simulink model "acdcmg_sim8_2_sc_gui"  (R2019b)
settings: Solver=ode8  StartTime=0.0  StopTime=0.5  FixedStep=4e-05  MaxStep=1e-2  RelTol=1e-3
PreLoadFcn:
  | Set_parameters_R2018
InitFcn:
  | Set_parameters_R2018
libraries: opal_lib x23
(part 1 of 2)
settings Model: ARTEMISmethode_block_infos=$$__separator__$$  Creator=Leony  LastModifiedBy=dkh20
settings SolverCC: ZeroCrossAlgorithm=Adaptive  SolverResetMethod=Robust
settings DataIOCC: LimitDataPoints=on  SaveFormat=Array  ReturnWorkspaceOutputs=off
settings OptimizationCC: LocalBlockOutputs=off  LifeSpan=inf
settings DebuggingCC: UnderspecifiedInitializationDetection=Classic  MergeDetectMultiDrivingBlocksExec=none  IgnoredZcDiagnostic=none  SolverPrmCheckMsg=warning  AllowSymbolicDim=off  SFUnexpectedBacktrackingDiag=warning  SFNoUnconditionalDefaultTransitionDiag=warning  SFExecutionAtInitializationDiag=none  ArithmeticOperatorsInVariantConditions=warning
settings HardwareCC: ProdBitPerPointer=32  ProdBitPerSizeT=32  ProdBitPerPtrDiffT=32  ProdLargestAtomicFloat=None  ProdIntDivRoundTo=Undefined  ProdEndianess=Unspecified  ProdWordSize=32  ProdHWDeviceType=32-bit Generic
settings ModelReferenceCC: PropagateSignalLabelsOutOfModel=off
settings SFSimCC: SimUseLocalCustomCode=off  CustomCodeUndefinedFunction=UseInterfaceOnly
settings RTWCC: GenCodeOnly=on  RTWUseLocalCustomCode=off
settings CodeAppCC: StateflowObjectComments=on
settings GRTTargetCC: TargetLangStandard=C89/C90 (ANSI)
settings ConfigComp: CovMetricSettings=dw  CovSaveCumulativeToWorkspaceVar=on  CovSaveSingleToWorkspaceVar=on  CovExternalEMLEnable=off
settings SimscapeCC: SimscapeNormalizeSystem=off

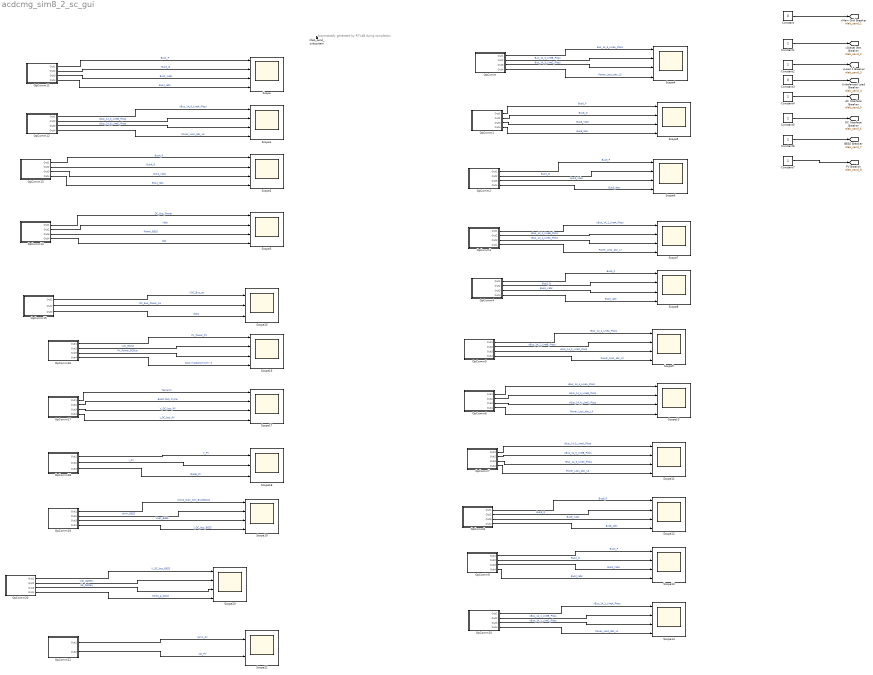
== system acdcmg_sim8_2_sc_gui ==
  note: Automatically generated by RT-LAB during compilation.
  Constant : Constant  Value=0
  Constant{1..2,4..7} (6 alike) : Constant
  Constant3 : Constant  Value=0
  OpComm : Subsystem
      mask init:
      | opmaskdisplay('maskdisplay_block',gcb,'disp(''OpComm'')');
      mask Display:
      | patch([0 0.5 0.7 0],[1 1 0 0],[0.7 0.75 0.9]);
      | patch([1 0.53 0.73 1],[1 1 0 0],[1 0.8 0.7]);
      | plot([0 0 1 1 0],[0 1 1 0 0]);
      | disp('OpComm')
  OpComm1 : Subsystem
      mask init:
      | opmaskdisplay('maskdisplay_block',gcb,'disp(''OpComm'')');
      mask Display:
      | patch([0 0.5 0.7 0],[1 1 0 0],[0.7 0.75 0.9]);
      | patch([1 0.53 0.73 1],[1 1 0 0],[1 0.8 0.7]);
      | plot([0 0 1 1 0],[0 1 1 0 0]);
      | disp('OpComm')
  OpComm10 : Subsystem
      mask init:
      | opmaskdisplay('maskdisplay_block',gcb,'disp(''OpComm'')');
      mask Display:
      | patch([0 0.5 0.7 0],[1 1 0 0],[0.7 0.75 0.9]);
      | patch([1 0.53 0.73 1],[1 1 0 0],[1 0.8 0.7]);
      | plot([0 0 1 1 0],[0 1 1 0 0]);
      | disp('OpComm')
  OpComm11 : Subsystem
      mask init:
      | opmaskdisplay('maskdisplay_block',gcb,'disp(''OpComm'')');
      mask Display:
      | patch([0 0.5 0.7 0],[1 1 0 0],[0.7 0.75 0.9]);
      | patch([1 0.53 0.73 1],[1 1 0 0],[1 0.8 0.7]);
      | plot([0 0 1 1 0],[0 1 1 0 0]);
      | disp('OpComm')
  OpComm12 : Subsystem
      mask init:
      | opmaskdisplay('maskdisplay_block',gcb,'disp(''OpComm'')');
      mask Display:
      | patch([0 0.5 0.7 0],[1 1 0 0],[0.7 0.75 0.9]);
      | patch([1 0.53 0.73 1],[1 1 0 0],[1 0.8 0.7]);
      | plot([0 0 1 1 0],[0 1 1 0 0]);
      | disp('OpComm')
  OpComm13 : Subsystem
      mask init:
      | opmaskdisplay('maskdisplay_block',gcb,'disp(''OpComm'')');
      mask Display:
      | patch([0 0.5 0.7 0],[1 1 0 0],[0.7 0.75 0.9]);
      | patch([1 0.53 0.73 1],[1 1 0 0],[1 0.8 0.7]);
      | plot([0 0 1 1 0],[0 1 1 0 0]);
      | disp('OpComm')
  OpComm14 : Subsystem
      mask init:
      | opmaskdisplay('maskdisplay_block',gcb,'disp(''OpComm'')');
      mask Display:
      | patch([0 0.5 0.7 0],[1 1 0 0],[0.7 0.75 0.9]);
      | patch([1 0.53 0.73 1],[1 1 0 0],[1 0.8 0.7]);
      | plot([0 0 1 1 0],[0 1 1 0 0]);
      | disp('OpComm')
  OpComm15 : Subsystem
      mask init:
      | opmaskdisplay('maskdisplay_block',gcb,'disp(''OpComm'')');
      mask Display:
      | patch([0 0.5 0.7 0],[1 1 0 0],[0.7 0.75 0.9]);
      | patch([1 0.53 0.73 1],[1 1 0 0],[1 0.8 0.7]);
      | plot([0 0 1 1 0],[0 1 1 0 0]);
      | disp('OpComm')
  OpComm16 : Subsystem
      mask init:
      | opmaskdisplay('maskdisplay_block',gcb,'disp(''OpComm'')');
      mask Display:
      | patch([0 0.5 0.7 0],[1 1 0 0],[0.7 0.75 0.9]);
      | patch([1 0.53 0.73 1],[1 1 0 0],[1 0.8 0.7]);
      | plot([0 0 1 1 0],[0 1 1 0 0]);
      | disp('OpComm')
  OpComm17 : Subsystem
      mask init:
      | opmaskdisplay('maskdisplay_block',gcb,'disp(''OpComm'')');
      mask Display:
      | patch([0 0.5 0.7 0],[1 1 0 0],[0.7 0.75 0.9]);
      | patch([1 0.53 0.73 1],[1 1 0 0],[1 0.8 0.7]);
      | plot([0 0 1 1 0],[0 1 1 0 0]);
      | disp('OpComm')
  OpComm18 : Subsystem
      mask init:
      | opmaskdisplay('maskdisplay_block',gcb,'disp(''OpComm'')');
      mask Display:
      | patch([0 0.5 0.7 0],[1 1 0 0],[0.7 0.75 0.9]);
      | patch([1 0.53 0.73 1],[1 1 0 0],[1 0.8 0.7]);
      | plot([0 0 1 1 0],[0 1 1 0 0]);
      | disp('OpComm')
  OpComm19 : Subsystem
      mask init:
      | opmaskdisplay('maskdisplay_block',gcb,'disp(''OpComm'')');
      mask Display:
      | patch([0 0.5 0.7 0],[1 1 0 0],[0.7 0.75 0.9]);
      | patch([1 0.53 0.73 1],[1 1 0 0],[1 0.8 0.7]);
      | plot([0 0 1 1 0],[0 1 1 0 0]);
      | disp('OpComm')
  OpComm2 : Subsystem
      mask init:
      | opmaskdisplay('maskdisplay_block',gcb,'disp(''OpComm'')');
      mask Display:
      | patch([0 0.5 0.7 0],[1 1 0 0],[0.7 0.75 0.9]);
      | patch([1 0.53 0.73 1],[1 1 0 0],[1 0.8 0.7]);
      | plot([0 0 1 1 0],[0 1 1 0 0]);
      | disp('OpComm')
  OpComm20 : Subsystem
      mask init:
      | opmaskdisplay('maskdisplay_block',gcb,'disp(''OpComm'')');
      mask Display:
      | patch([0 0.5 0.7 0],[1 1 0 0],[0.7 0.75 0.9]);
      | patch([1 0.53 0.73 1],[1 1 0 0],[1 0.8 0.7]);
      | plot([0 0 1 1 0],[0 1 1 0 0]);
      | disp('OpComm')
  OpComm21 : Subsystem
      mask init:
      | opmaskdisplay('maskdisplay_block',gcb,'disp(''OpComm'')');
      mask Display:
      | patch([0 0.5 0.7 0],[1 1 0 0],[0.7 0.75 0.9]);
      | patch([1 0.53 0.73 1],[1 1 0 0],[1 0.8 0.7]);
      | plot([0 0 1 1 0],[0 1 1 0 0]);
      | disp('OpComm')
  OpComm3 : Subsystem
      mask init:
      | opmaskdisplay('maskdisplay_block',gcb,'disp(''OpComm'')');
      mask Display:
      | patch([0 0.5 0.7 0],[1 1 0 0],[0.7 0.75 0.9]);
      | patch([1 0.53 0.73 1],[1 1 0 0],[1 0.8 0.7]);
      | plot([0 0 1 1 0],[0 1 1 0 0]);
      | disp('OpComm')
  OpComm4 : Subsystem
      mask init:
      | opmaskdisplay('maskdisplay_block',gcb,'disp(''OpComm'')');
      mask Display:
      | patch([0 0.5 0.7 0],[1 1 0 0],[0.7 0.75 0.9]);
      | patch([1 0.53 0.73 1],[1 1 0 0],[1 0.8 0.7]);
      | plot([0 0 1 1 0],[0 1 1 0 0]);
      | disp('OpComm')
  OpComm5 : Subsystem
      mask init:
      | opmaskdisplay('maskdisplay_block',gcb,'disp(''OpComm'')');
      mask Display:
      | patch([0 0.5 0.7 0],[1 1 0 0],[0.7 0.75 0.9]);
      | patch([1 0.53 0.73 1],[1 1 0 0],[1 0.8 0.7]);
      | plot([0 0 1 1 0],[0 1 1 0 0]);
      | disp('OpComm')
  OpComm6 : Subsystem
      mask init:
      | opmaskdisplay('maskdisplay_block',gcb,'disp(''OpComm'')');
      mask Display:
      | patch([0 0.5 0.7 0],[1 1 0 0],[0.7 0.75 0.9]);
      | patch([1 0.53 0.73 1],[1 1 0 0],[1 0.8 0.7]);
      | plot([0 0 1 1 0],[0 1 1 0 0]);
      | disp('OpComm')
  OpComm7 : Subsystem
      mask init:
      | opmaskdisplay('maskdisplay_block',gcb,'disp(''OpComm'')');
      mask Display:
      | patch([0 0.5 0.7 0],[1 1 0 0],[0.7 0.75 0.9]);
      | patch([1 0.53 0.73 1],[1 1 0 0],[1 0.8 0.7]);
      | plot([0 0 1 1 0],[0 1 1 0 0]);
      | disp('OpComm')
  OpComm8 : Subsystem
      mask init:
      | opmaskdisplay('maskdisplay_block',gcb,'disp(''OpComm'')');
      mask Display:
      | patch([0 0.5 0.7 0],[1 1 0 0],[0.7 0.75 0.9]);
      | patch([1 0.53 0.73 1],[1 1 0 0],[1 0.8 0.7]);
      | plot([0 0 1 1 0],[0 1 1 0 0]);
      | disp('OpComm')
  OpComm9 : Subsystem
      mask init:
      | opmaskdisplay('maskdisplay_block',gcb,'disp(''OpComm'')');
      mask Display:
      | patch([0 0.5 0.7 0],[1 1 0 0],[0.7 0.75 0.9]);
      | patch([1 0.53 0.73 1],[1 1 0 0],[1 0.8 0.7]);
      | plot([0 0 1 1 0],[0 1 1 0 0]);
      | disp('OpComm')
  Scope{,1..14,16..17,19..20} (19 alike) : Scope  NumInputPorts=4
  Scope15 : Scope  NumInputPorts=3
  Scope18 : Scope  NumInputPorts=3
  Scope21 : Scope  NumInputPorts=2
  rtlab_send_subsystem : Subsystem  Priority=-100
      mask Display: text(0,0,'');
  tag scope: rtlab_send_1=global, rtlab_send_2=global, rtlab_send_3=global, rtlab_send_4=global, rtlab_send_5=global, rtlab_send_6=global, rtlab_send_7=global, rtlab_send_8=global
  wires:
  OpComm21/2(Out2) -> Scope21/2  "Idc_PV"
  OpComm21/1(Out1) -> Scope21/1  "Iprim_PV"
  OpComm20/4(Out4) -> Scope20/4  "Comp_g_boost"
  OpComm20/3(Out3) -> Scope20/3  "Idc_battery"
  OpComm20/2(Out2) -> Scope20/2  "Vdc_battery"
  OpComm20/1(Out1) -> Scope20/1  "V_DC_bus_BESS"
  OpComm19/4(Out4) -> Scope19/4  "I_DC_bus_BESS"
  OpComm19/3(Out3) -> Scope19/3  "Vsec_BESS"
  OpComm19/2(Out2) -> Scope19/2  "Iprim_BESS"
  OpComm19/1(Out1) -> Scope19/1  "Comp_Duty_Ctrl_BuckBoost"
  OpComm18/3(Out3) -> Scope18/3  "Idiode_PV"
  OpComm18/2(Out2) -> Scope18/2  "I_PV"
  OpComm18/1(Out1) -> Scope18/1  "V_PV"
  OpComm17/4(Out4) -> Scope17/4  "I_DC_bus_PV"
  OpComm17/3(Out3) -> Scope17/3  "V_DC_bus_PV"
  OpComm17/2(Out2) -> Scope17/2  "Boost Duty Cycle"
  OpComm17/1(Out1) -> Scope17/1  "Temp(C)"
  OpComm16/4(Out4) -> Scope16/4  "Solar Irradiance W/m^2"
  OpComm16/3(Out3) -> Scope16/3  "PV_Power_DCBus"
  OpComm16/2(Out2) -> Scope16/2  "Vdc_Boost"
  OpComm16/1(Out1) -> Scope16/1  "PV_Power_PV"
  OpComm15/3(Out3) -> Scope15/3  "Ibat1"
  OpComm15/2(Out2) -> Scope15/2  "DC_Bus_Power_kw"
  OpComm15/1(Out1) -> Scope15/1  "VDC_Bus_pu"
  OpComm14/4(Out4) -> Scope3/4  "Ibat"
  OpComm14/3(Out3) -> Scope3/3  "Power_BESS"
  OpComm14/2(Out2) -> Scope3/2  "Vbat"
  OpComm14/1(Out1) -> Scope3/1  "DC_Bus_Power"
  OpComm13/4(Out4) -> Scope2/4  "Bus4_Iabc"
  OpComm13/3(Out3) -> Scope2/3  "Bus4_Vabc"
  OpComm13/2(Out2) -> Scope2/2  "Bus4_Q"
  OpComm13/1(Out1) -> Scope2/1  "Bus4_P"
  OpComm12/4(Out4) -> Scope1/4  "Power_Loss_abc_L6"
  OpComm12/3(Out3) -> Scope1/3  "xBus_14_6_LineC_Ploss"
  OpComm12/2(Out2) -> Scope1/2  "xBus_14_6_LineB_Ploss"
  OpComm12/1(Out1) -> Scope1/1  "xBus_14_6_LineA_Ploss"
  OpComm11/4(Out4) -> Scope/4  "Bus1_Iabc"
  OpComm11/3(Out3) -> Scope/3  "Bus1_Vabc"
  OpComm11/2(Out2) -> Scope/2  "Bus1_Q"
  OpComm11/1(Out1) -> Scope/1  "Bus1_P"
  OpComm9/4(Out4) -> Scope13/4  "Bus2_Iabc"
  OpComm9/3(Out3) -> Scope13/3  "Bus2_Vabc"
  OpComm9/2(Out2) -> Scope13/2  "Bus2_Q"
  OpComm9/1(Out1) -> Scope13/1  "Bus2_P"
  OpComm10/4(Out4) -> Scope14/4  "Power_Loss_abc_L1"
  OpComm10/3(Out3) -> Scope14/3  "xBus_14_1_LineC_Ploss"
  OpComm10/2(Out2) -> Scope14/2  "xBus_14_1_LineB_Ploss"
  OpComm10/1(Out1) -> Scope14/1  "xBus_14_1_LineA_Ploss"
  OpComm8/4(Out4) -> Scope12/4  "Bus8_Iabc"
  OpComm8/3(Out3) -> Scope12/3  "Bus8_Vabc"
  OpComm8/2(Out2) -> Scope12/2  "Bus8_Q"
  OpComm8/1(Out1) -> Scope12/1  "Bus8_P"
  OpComm7/4(Out4) -> Scope11/4  "Power_Loss_abc_L5"
  OpComm7/3(Out3) -> Scope11/3  "xBus_14_5_LineC_Ploss"
  OpComm7/2(Out2) -> Scope11/2  "xBus_14_5_LineB_Ploss"
  OpComm7/1(Out1) -> Scope11/1  "xBus_14_5_LineA_Ploss"
  OpComm6/4(Out4) -> Scope10/4  "Power_Loss_abc_L4"
  OpComm6/3(Out3) -> Scope10/3  "xBus_14_4_LineC_Ploss"
  OpComm6/2(Out2) -> Scope10/2  "xBus_14_4_LineB_Ploss"
  OpComm6/1(Out1) -> Scope10/1  "xBus_14_4_LineA_Ploss"
  OpComm5/4(Out4) -> Scope9/4  "Power_Loss_abc_L2"
  OpComm5/3(Out3) -> Scope9/3  "xBus_14_2_LineC_Ploss"
  OpComm5/2(Out2) -> Scope9/2  "xBus_14_2_LineB_Ploss"
  OpComm5/1(Out1) -> Scope9/1  "xBus_14_2_LineA_Ploss"
  OpComm4/1(Out1) -> Scope8/1  "Bus5_P"
  OpComm4/4(Out4) -> Scope8/4  "Bus5_Iabc"
  OpComm4/3(Out3) -> Scope8/3  "Bus5_Vabc"
  OpComm4/2(Out2) -> Scope8/2  "Bus5_Q"
  OpComm3/4(Out4) -> Scope7/4  "Power_Loss_abc_L7"
  OpComm3/1(Out1) -> Scope7/1  "xBus_14_1_LineA_Ploss"
  OpComm3/3(Out3) -> Scope7/3  "xBus_14_1_LineC_Ploss"
  OpComm3/2(Out2) -> Scope7/2  "xBus_14_1_LineB_Ploss"
  OpComm2/4(Out4) -> Scope6/4  "Bus3_Iabc"
  OpComm2/3(Out3) -> Scope6/3  "Bus3_Vabc"
  OpComm2/2(Out2) -> Scope6/2  "Bus3_Q"
  OpComm2/1(Out1) -> Scope6/1  "Bus3_P"
  OpComm1/4(Out4) -> Scope5/4  "Bus6_Iabc"
  OpComm1/1(Out1) -> Scope5/1  "Bus6_P"
  OpComm1/3(Out3) -> Scope5/3  "Bus6_Vabc"
  OpComm1/2(Out2) -> Scope5/2  "Bus6_Q"
  OpComm/4(Out4) -> Scope4/4  "Power_Loss_abc_L3"
  OpComm/3(Out3) -> Scope4/3  "Bus_14_3_LineC_Ploss"
  OpComm/2(Out2) -> Scope4/2  "Bus_14_3_LineB_Ploss"
  OpComm/1(Out1) -> Scope4/1  "Bus_14_3_LineA_Ploss"
  Constant7/1 -> [rtlab_send_8]
  Constant6/1 -> [rtlab_send_7]
  Constant5/1 -> [rtlab_send_6]
  Constant4/1 -> [rtlab_send_5]
  Constant3/1 -> [rtlab_send_4]
  Constant2/1 -> [rtlab_send_3]
  Constant1/1 -> [rtlab_send_2]
  Constant/1 -> [rtlab_send_1]

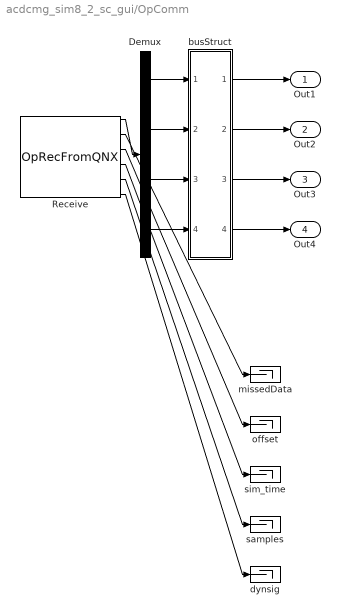
== system acdcmg_sim8_2_sc_gui/OpComm ==
  Demux : Demux  Outputs="[1  1  1  3]"
  Receive : opal_lib/Communication/OpRecFromQNX  Node_num=1  Acqu_Group=1  Data_Width=6  Synchronization=on  Interpolation=on  Threshold=1.0  modelname=ACDCMG_sim8.slx  sampletime=4e-05
  busStruct : Subsystem
  dynsig : Terminator
  missedData : Terminator
  offset : Terminator
  samples : Terminator
  sim_time : Terminator
  Out1 : Outport
  Out2 : Outport  Port=2
  Out3 : Outport  Port=3
  Out4 : Outport  Port=4
  wires:
  Demux/4 -> busStruct/4(In4)
  Demux/3 -> busStruct/3(In3)
  Demux/2 -> busStruct/2(In2)
  Demux/1 -> busStruct/1(In1)
  busStruct/4(Out4) -> Out4/1
  busStruct/3(Out3) -> Out3/1
  busStruct/2(Out2) -> Out2/1
  busStruct/1(Out1) -> Out1/1
  Receive/1 -> Demux/1
  Receive/6 -> dynsig/1
  Receive/5 -> samples/1
  Receive/4 -> sim_time/1
  Receive/3 -> offset/1
  Receive/2 -> missedData/1

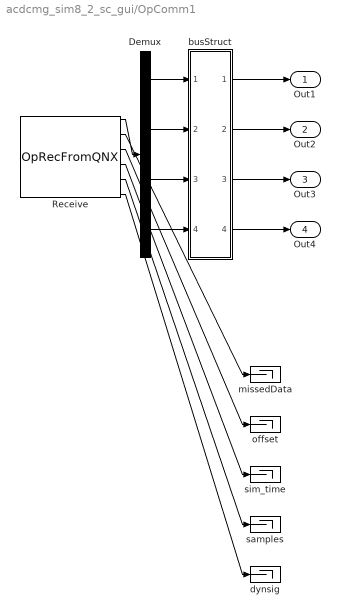
== system acdcmg_sim8_2_sc_gui/OpComm1 ==
  Demux : Demux  Outputs="[1  1  3  3]"
  Receive : opal_lib/Communication/OpRecFromQNX  Node_num=1  Acqu_Group=2  Data_Width=8  Synchronization=on  Interpolation=on  Threshold=1.0  modelname=ACDCMG_sim8.slx  sampletime=4e-05
  busStruct : Subsystem
  dynsig : Terminator
  missedData : Terminator
  offset : Terminator
  samples : Terminator
  sim_time : Terminator
  Out1 : Outport
  Out2 : Outport  Port=2
  Out3 : Outport  Port=3
  Out4 : Outport  Port=4
  wires:
  Demux/4 -> busStruct/4(In4)
  Demux/3 -> busStruct/3(In3)
  Demux/2 -> busStruct/2(In2)
  Demux/1 -> busStruct/1(In1)
  busStruct/4(Out4) -> Out4/1
  busStruct/3(Out3) -> Out3/1
  busStruct/2(Out2) -> Out2/1
  busStruct/1(Out1) -> Out1/1
  Receive/1 -> Demux/1
  Receive/6 -> dynsig/1
  Receive/5 -> samples/1
  Receive/4 -> sim_time/1
  Receive/3 -> offset/1
  Receive/2 -> missedData/1

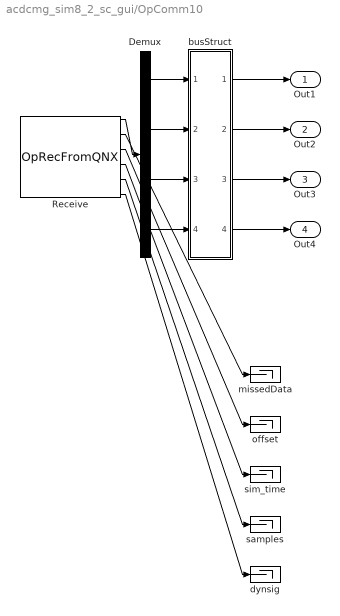
== system acdcmg_sim8_2_sc_gui/OpComm10 ==
  Demux : Demux  Outputs="[1  1  1  3]"
  Receive : opal_lib/Communication/OpRecFromQNX  Node_num=1  Acqu_Group=11  Data_Width=6  Synchronization=on  Interpolation=on  Threshold=1.0  modelname=ACDCMG_sim8.slx  sampletime=4e-05
  busStruct : Subsystem
  dynsig : Terminator
  missedData : Terminator
  offset : Terminator
  samples : Terminator
  sim_time : Terminator
  Out1 : Outport
  Out2 : Outport  Port=2
  Out3 : Outport  Port=3
  Out4 : Outport  Port=4
  wires:
  Demux/4 -> busStruct/4(In4)
  Demux/3 -> busStruct/3(In3)
  Demux/2 -> busStruct/2(In2)
  Demux/1 -> busStruct/1(In1)
  busStruct/4(Out4) -> Out4/1
  busStruct/3(Out3) -> Out3/1
  busStruct/2(Out2) -> Out2/1
  busStruct/1(Out1) -> Out1/1
  Receive/1 -> Demux/1
  Receive/6 -> dynsig/1
  Receive/5 -> samples/1
  Receive/4 -> sim_time/1
  Receive/3 -> offset/1
  Receive/2 -> missedData/1

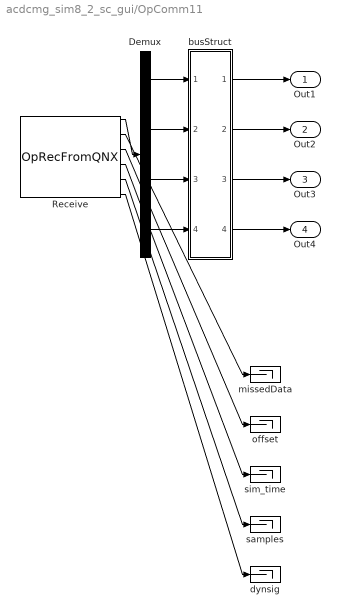
== system acdcmg_sim8_2_sc_gui/OpComm11 ==
  Demux : Demux  Outputs="[1  1  3  3]"
  Receive : opal_lib/Communication/OpRecFromQNX  Node_num=1  Acqu_Group=12  Data_Width=8  Synchronization=on  Interpolation=on  Threshold=1.0  modelname=ACDCMG_sim8.slx  sampletime=4e-05
  busStruct : Subsystem
  dynsig : Terminator
  missedData : Terminator
  offset : Terminator
  samples : Terminator
  sim_time : Terminator
  Out1 : Outport
  Out2 : Outport  Port=2
  Out3 : Outport  Port=3
  Out4 : Outport  Port=4
  wires:
  Demux/4 -> busStruct/4(In4)
  Demux/3 -> busStruct/3(In3)
  Demux/2 -> busStruct/2(In2)
  Demux/1 -> busStruct/1(In1)
  busStruct/4(Out4) -> Out4/1
  busStruct/3(Out3) -> Out3/1
  busStruct/2(Out2) -> Out2/1
  busStruct/1(Out1) -> Out1/1
  Receive/1 -> Demux/1
  Receive/6 -> dynsig/1
  Receive/5 -> samples/1
  Receive/4 -> sim_time/1
  Receive/3 -> offset/1
  Receive/2 -> missedData/1

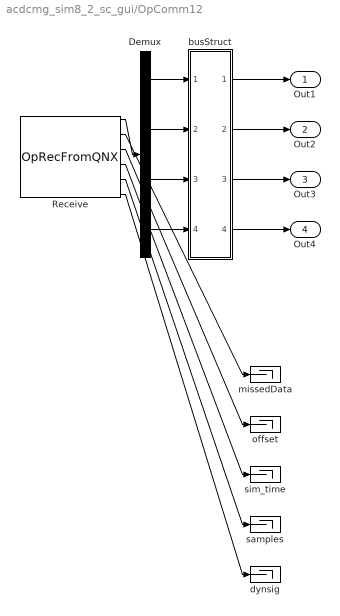
== system acdcmg_sim8_2_sc_gui/OpComm12 ==
  Demux : Demux  Outputs="[1  1  1  3]"
  Receive : opal_lib/Communication/OpRecFromQNX  Node_num=1  Acqu_Group=13  Data_Width=6  Synchronization=on  Interpolation=on  Threshold=1.0  modelname=ACDCMG_sim8.slx  sampletime=4e-05
  busStruct : Subsystem
  dynsig : Terminator
  missedData : Terminator
  offset : Terminator
  samples : Terminator
  sim_time : Terminator
  Out1 : Outport
  Out2 : Outport  Port=2
  Out3 : Outport  Port=3
  Out4 : Outport  Port=4
  wires:
  Demux/4 -> busStruct/4(In4)
  Demux/3 -> busStruct/3(In3)
  Demux/2 -> busStruct/2(In2)
  Demux/1 -> busStruct/1(In1)
  busStruct/4(Out4) -> Out4/1
  busStruct/3(Out3) -> Out3/1
  busStruct/2(Out2) -> Out2/1
  busStruct/1(Out1) -> Out1/1
  Receive/1 -> Demux/1
  Receive/6 -> dynsig/1
  Receive/5 -> samples/1
  Receive/4 -> sim_time/1
  Receive/3 -> offset/1
  Receive/2 -> missedData/1

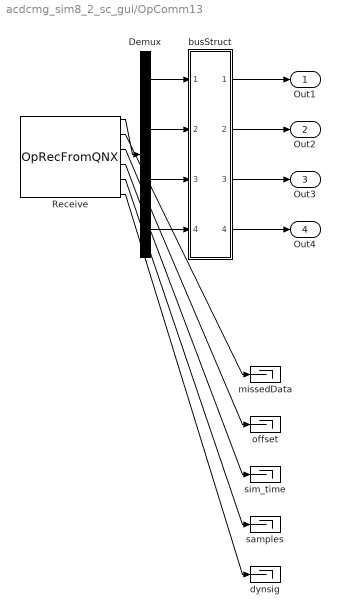
== system acdcmg_sim8_2_sc_gui/OpComm13 ==
  Demux : Demux  Outputs="[1  1  3  3]"
  Receive : opal_lib/Communication/OpRecFromQNX  Node_num=1  Acqu_Group=14  Data_Width=8  Synchronization=on  Interpolation=on  Threshold=1.0  modelname=ACDCMG_sim8.slx  sampletime=4e-05
  busStruct : Subsystem
  dynsig : Terminator
  missedData : Terminator
  offset : Terminator
  samples : Terminator
  sim_time : Terminator
  Out1 : Outport
  Out2 : Outport  Port=2
  Out3 : Outport  Port=3
  Out4 : Outport  Port=4
  wires:
  Demux/4 -> busStruct/4(In4)
  Demux/3 -> busStruct/3(In3)
  Demux/2 -> busStruct/2(In2)
  Demux/1 -> busStruct/1(In1)
  busStruct/4(Out4) -> Out4/1
  busStruct/3(Out3) -> Out3/1
  busStruct/2(Out2) -> Out2/1
  busStruct/1(Out1) -> Out1/1
  Receive/1 -> Demux/1
  Receive/6 -> dynsig/1
  Receive/5 -> samples/1
  Receive/4 -> sim_time/1
  Receive/3 -> offset/1
  Receive/2 -> missedData/1

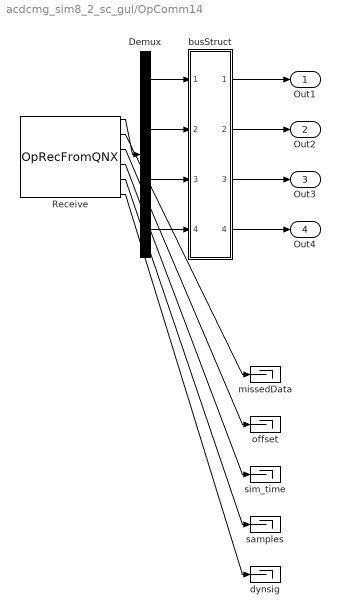
== system acdcmg_sim8_2_sc_gui/OpComm14 ==
  Demux : Demux  Outputs="[1  1  1  1]"
  Receive : opal_lib/Communication/OpRecFromQNX  Node_num=1  Acqu_Group=16  Data_Width=4  Synchronization=on  Interpolation=on  Threshold=1.0  modelname=ACDCMG_sim8.slx  sampletime=4e-05
  busStruct : Subsystem
  dynsig : Terminator
  missedData : Terminator
  offset : Terminator
  samples : Terminator
  sim_time : Terminator
  Out1 : Outport
  Out2 : Outport  Port=2
  Out3 : Outport  Port=3
  Out4 : Outport  Port=4
  wires:
  Demux/4 -> busStruct/4(In4)
  Demux/3 -> busStruct/3(In3)
  Demux/2 -> busStruct/2(In2)
  Demux/1 -> busStruct/1(In1)
  busStruct/4(Out4) -> Out4/1
  busStruct/3(Out3) -> Out3/1
  busStruct/2(Out2) -> Out2/1
  busStruct/1(Out1) -> Out1/1
  Receive/1 -> Demux/1
  Receive/6 -> dynsig/1
  Receive/5 -> samples/1
  Receive/4 -> sim_time/1
  Receive/3 -> offset/1
  Receive/2 -> missedData/1

== system acdcmg_sim8_2_sc_gui/OpComm15 ==
  Demux : Demux  Outputs="[1  1  1]"
  Receive : opal_lib/Communication/OpRecFromQNX  Node_num=1  Acqu_Group=17  Data_Width=3  Synchronization=on  Interpolation=on  Threshold=1.0  modelname=ACDCMG_sim8.slx  sampletime=4e-05
  busStruct : Subsystem
  dynsig : Terminator
  missedData : Terminator
  offset : Terminator
  samples : Terminator
  sim_time : Terminator
  Out1 : Outport
  Out2 : Outport  Port=2
  Out3 : Outport  Port=3
  wires:
  Demux/3 -> busStruct/3(In3)
  Demux/2 -> busStruct/2(In2)
  Demux/1 -> busStruct/1(In1)
  busStruct/3(Out3) -> Out3/1
  busStruct/2(Out2) -> Out2/1
  busStruct/1(Out1) -> Out1/1
  Receive/1 -> Demux/1
  Receive/6 -> dynsig/1
  Receive/5 -> samples/1
  Receive/4 -> sim_time/1
  Receive/3 -> offset/1
  Receive/2 -> missedData/1

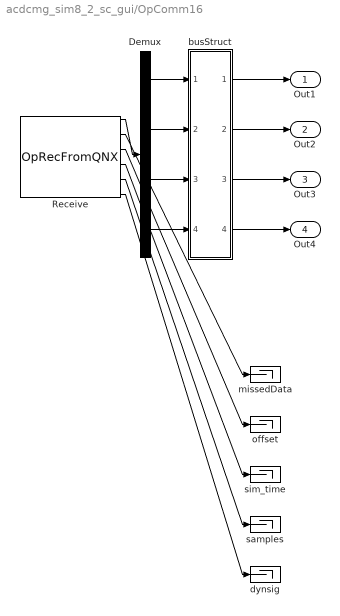
== system acdcmg_sim8_2_sc_gui/OpComm16 ==
  Demux : Demux  Outputs="[1  1  1  1]"
  Receive : opal_lib/Communication/OpRecFromQNX  Node_num=1  Acqu_Group=18  Data_Width=4  Synchronization=on  Interpolation=on  Threshold=1.0  modelname=ACDCMG_sim8.slx  sampletime=4e-05
  busStruct : Subsystem
  dynsig : Terminator
  missedData : Terminator
  offset : Terminator
  samples : Terminator
  sim_time : Terminator
  Out1 : Outport
  Out2 : Outport  Port=2
  Out3 : Outport  Port=3
  Out4 : Outport  Port=4
  wires:
  Demux/4 -> busStruct/4(In4)
  Demux/3 -> busStruct/3(In3)
  Demux/2 -> busStruct/2(In2)
  Demux/1 -> busStruct/1(In1)
  busStruct/4(Out4) -> Out4/1
  busStruct/3(Out3) -> Out3/1
  busStruct/2(Out2) -> Out2/1
  busStruct/1(Out1) -> Out1/1
  Receive/1 -> Demux/1
  Receive/6 -> dynsig/1
  Receive/5 -> samples/1
  Receive/4 -> sim_time/1
  Receive/3 -> offset/1
  Receive/2 -> missedData/1

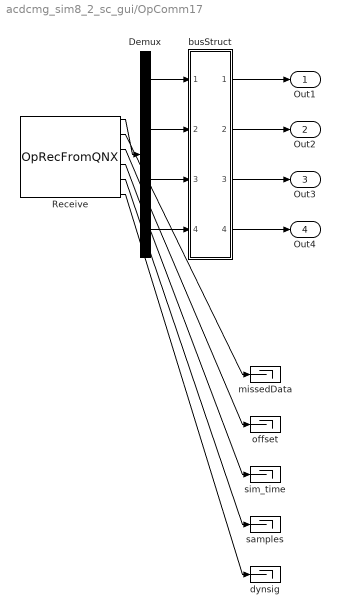
== system acdcmg_sim8_2_sc_gui/OpComm17 ==
  Demux : Demux  Outputs="[1  1  1  1]"
  Receive : opal_lib/Communication/OpRecFromQNX  Node_num=1  Acqu_Group=19  Data_Width=4  Synchronization=on  Interpolation=on  Threshold=1.0  modelname=ACDCMG_sim8.slx  sampletime=4e-05
  busStruct : Subsystem
  dynsig : Terminator
  missedData : Terminator
  offset : Terminator
  samples : Terminator
  sim_time : Terminator
  Out1 : Outport
  Out2 : Outport  Port=2
  Out3 : Outport  Port=3
  Out4 : Outport  Port=4
  wires:
  Demux/4 -> busStruct/4(In4)
  Demux/3 -> busStruct/3(In3)
  Demux/2 -> busStruct/2(In2)
  Demux/1 -> busStruct/1(In1)
  busStruct/4(Out4) -> Out4/1
  busStruct/3(Out3) -> Out3/1
  busStruct/2(Out2) -> Out2/1
  busStruct/1(Out1) -> Out1/1
  Receive/1 -> Demux/1
  Receive/6 -> dynsig/1
  Receive/5 -> samples/1
  Receive/4 -> sim_time/1
  Receive/3 -> offset/1
  Receive/2 -> missedData/1

== system acdcmg_sim8_2_sc_gui/OpComm18 ==
  Demux : Demux  Outputs="[1  1  1]"
  Receive : opal_lib/Communication/OpRecFromQNX  Node_num=1  Acqu_Group=20  Data_Width=3  Synchronization=on  Interpolation=on  Threshold=1.0  modelname=ACDCMG_sim8.slx  sampletime=4e-05
  busStruct : Subsystem
  dynsig : Terminator
  missedData : Terminator
  offset : Terminator
  samples : Terminator
  sim_time : Terminator
  Out1 : Outport
  Out2 : Outport  Port=2
  Out3 : Outport  Port=3
  wires:
  Demux/3 -> busStruct/3(In3)
  Demux/2 -> busStruct/2(In2)
  Demux/1 -> busStruct/1(In1)
  busStruct/3(Out3) -> Out3/1
  busStruct/2(Out2) -> Out2/1
  busStruct/1(Out1) -> Out1/1
  Receive/1 -> Demux/1
  Receive/6 -> dynsig/1
  Receive/5 -> samples/1
  Receive/4 -> sim_time/1
  Receive/3 -> offset/1
  Receive/2 -> missedData/1

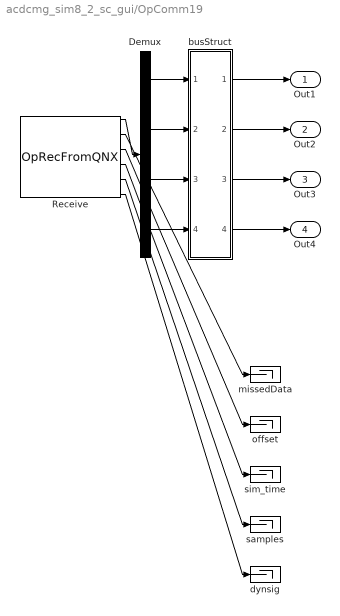
== system acdcmg_sim8_2_sc_gui/OpComm19 ==
  Demux : Demux  Outputs="[1  1  1  1]"
  Receive : opal_lib/Communication/OpRecFromQNX  Node_num=1  Acqu_Group=21  Data_Width=4  Synchronization=on  Interpolation=on  Threshold=1.0  modelname=ACDCMG_sim8.slx  sampletime=4e-05
  busStruct : Subsystem
  dynsig : Terminator
  missedData : Terminator
  offset : Terminator
  samples : Terminator
  sim_time : Terminator
  Out1 : Outport
  Out2 : Outport  Port=2
  Out3 : Outport  Port=3
  Out4 : Outport  Port=4
  wires:
  Demux/4 -> busStruct/4(In4)
  Demux/3 -> busStruct/3(In3)
  Demux/2 -> busStruct/2(In2)
  Demux/1 -> busStruct/1(In1)
  busStruct/4(Out4) -> Out4/1
  busStruct/3(Out3) -> Out3/1
  busStruct/2(Out2) -> Out2/1
  busStruct/1(Out1) -> Out1/1
  Receive/1 -> Demux/1
  Receive/6 -> dynsig/1
  Receive/5 -> samples/1
  Receive/4 -> sim_time/1
  Receive/3 -> offset/1
  Receive/2 -> missedData/1

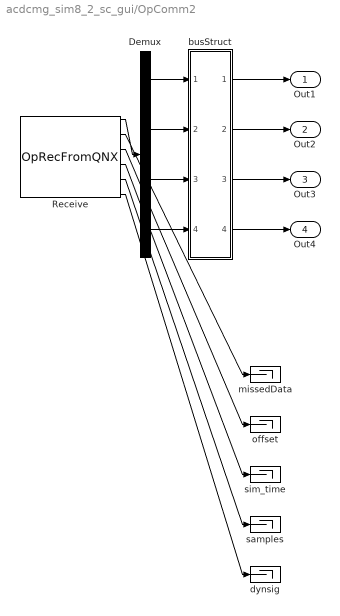
== system acdcmg_sim8_2_sc_gui/OpComm2 ==
  Demux : Demux  Outputs="[1  1  3  3]"
  Receive : opal_lib/Communication/OpRecFromQNX  Node_num=1  Acqu_Group=3  Data_Width=8  Synchronization=on  Interpolation=on  Threshold=1.0  modelname=ACDCMG_sim8.slx  sampletime=4e-05
  busStruct : Subsystem
  dynsig : Terminator
  missedData : Terminator
  offset : Terminator
  samples : Terminator
  sim_time : Terminator
  Out1 : Outport
  Out2 : Outport  Port=2
  Out3 : Outport  Port=3
  Out4 : Outport  Port=4
  wires:
  Demux/4 -> busStruct/4(In4)
  Demux/3 -> busStruct/3(In3)
  Demux/2 -> busStruct/2(In2)
  Demux/1 -> busStruct/1(In1)
  busStruct/4(Out4) -> Out4/1
  busStruct/3(Out3) -> Out3/1
  busStruct/2(Out2) -> Out2/1
  busStruct/1(Out1) -> Out1/1
  Receive/1 -> Demux/1
  Receive/6 -> dynsig/1
  Receive/5 -> samples/1
  Receive/4 -> sim_time/1
  Receive/3 -> offset/1
  Receive/2 -> missedData/1

== system acdcmg_sim8_2_sc_gui/OpComm20 ==
  Demux : Demux  Outputs="[1  1  1  1]"
  Receive : opal_lib/Communication/OpRecFromQNX  Node_num=1  Acqu_Group=22  Data_Width=4  Synchronization=on  Interpolation=on  Threshold=1.0  modelname=ACDCMG_sim8.slx  sampletime=4e-05
  busStruct : Subsystem
  dynsig : Terminator
  missedData : Terminator
  offset : Terminator
  samples : Terminator
  sim_time : Terminator
  Out1 : Outport
  Out2 : Outport  Port=2
  Out3 : Outport  Port=3
  Out4 : Outport  Port=4
  wires:
  Demux/4 -> busStruct/4(In4)
  Demux/3 -> busStruct/3(In3)
  Demux/2 -> busStruct/2(In2)
  Demux/1 -> busStruct/1(In1)
  busStruct/4(Out4) -> Out4/1
  busStruct/3(Out3) -> Out3/1
  busStruct/2(Out2) -> Out2/1
  busStruct/1(Out1) -> Out1/1
  Receive/1 -> Demux/1
  Receive/6 -> dynsig/1
  Receive/5 -> samples/1
  Receive/4 -> sim_time/1
  Receive/3 -> offset/1
  Receive/2 -> missedData/1

== system acdcmg_sim8_2_sc_gui/OpComm21 ==
  Demux : Demux  Outputs="[1  1]"
  Receive : opal_lib/Communication/OpRecFromQNX  Node_num=1  Acqu_Group=23  Data_Width=2  Synchronization=on  Interpolation=on  Threshold=1.0  modelname=ACDCMG_sim8.slx  sampletime=4e-05
  busStruct : Subsystem
  dynsig : Terminator
  missedData : Terminator
  offset : Terminator
  samples : Terminator
  sim_time : Terminator
  Out1 : Outport
  Out2 : Outport  Port=2
  wires:
  Demux/2 -> busStruct/2(In2)
  Demux/1 -> busStruct/1(In1)
  busStruct/2(Out2) -> Out2/1
  busStruct/1(Out1) -> Out1/1
  Receive/1 -> Demux/1
  Receive/6 -> dynsig/1
  Receive/5 -> samples/1
  Receive/4 -> sim_time/1
  Receive/3 -> offset/1
  Receive/2 -> missedData/1

== system acdcmg_sim8_2_sc_gui/OpComm3 ==
  Demux : Demux  Outputs="[1  1  1  3]"
  Receive : opal_lib/Communication/OpRecFromQNX  Node_num=1  Acqu_Group=4  Data_Width=6  Synchronization=on  Interpolation=on  Threshold=1.0  modelname=ACDCMG_sim8.slx  sampletime=4e-05
  busStruct : Subsystem
  dynsig : Terminator
  missedData : Terminator
  offset : Terminator
  samples : Terminator
  sim_time : Terminator
  Out1 : Outport
  Out2 : Outport  Port=2
  Out3 : Outport  Port=3
  Out4 : Outport  Port=4
  wires:
  Demux/4 -> busStruct/4(In4)
  Demux/3 -> busStruct/3(In3)
  Demux/2 -> busStruct/2(In2)
  Demux/1 -> busStruct/1(In1)
  busStruct/4(Out4) -> Out4/1
  busStruct/3(Out3) -> Out3/1
  busStruct/2(Out2) -> Out2/1
  busStruct/1(Out1) -> Out1/1
  Receive/1 -> Demux/1
  Receive/6 -> dynsig/1
  Receive/5 -> samples/1
  Receive/4 -> sim_time/1
  Receive/3 -> offset/1
  Receive/2 -> missedData/1

== system acdcmg_sim8_2_sc_gui/OpComm4 ==
  Demux : Demux  Outputs="[1  1  4  3]"
  Receive : opal_lib/Communication/OpRecFromQNX  Node_num=1  Acqu_Group=5  Data_Width=9  Synchronization=on  Interpolation=on  Threshold=1.0  modelname=ACDCMG_sim8.slx  sampletime=4e-05
  busStruct : Subsystem
  dynsig : Terminator
  missedData : Terminator
  offset : Terminator
  samples : Terminator
  sim_time : Terminator
  Out1 : Outport
  Out2 : Outport  Port=2
  Out3 : Outport  Port=3
  Out4 : Outport  Port=4
  wires:
  Demux/4 -> busStruct/4(In4)
  Demux/3 -> busStruct/3(In3)
  Demux/2 -> busStruct/2(In2)
  Demux/1 -> busStruct/1(In1)
  busStruct/4(Out4) -> Out4/1
  busStruct/3(Out3) -> Out3/1
  busStruct/2(Out2) -> Out2/1
  busStruct/1(Out1) -> Out1/1
  Receive/1 -> Demux/1
  Receive/6 -> dynsig/1
  Receive/5 -> samples/1
  Receive/4 -> sim_time/1
  Receive/3 -> offset/1
  Receive/2 -> missedData/1

== system acdcmg_sim8_2_sc_gui/OpComm5 ==
  Demux : Demux  Outputs="[1  1  1  3]"
  Receive : opal_lib/Communication/OpRecFromQNX  Node_num=1  Acqu_Group=6  Data_Width=6  Synchronization=on  Interpolation=on  Threshold=1.0  modelname=ACDCMG_sim8.slx  sampletime=4e-05
  busStruct : Subsystem
  dynsig : Terminator
  missedData : Terminator
  offset : Terminator
  samples : Terminator
  sim_time : Terminator
  Out1 : Outport
  Out2 : Outport  Port=2
  Out3 : Outport  Port=3
  Out4 : Outport  Port=4
  wires:
  Demux/4 -> busStruct/4(In4)
  Demux/3 -> busStruct/3(In3)
  Demux/2 -> busStruct/2(In2)
  Demux/1 -> busStruct/1(In1)
  busStruct/4(Out4) -> Out4/1
  busStruct/3(Out3) -> Out3/1
  busStruct/2(Out2) -> Out2/1
  busStruct/1(Out1) -> Out1/1
  Receive/1 -> Demux/1
  Receive/6 -> dynsig/1
  Receive/5 -> samples/1
  Receive/4 -> sim_time/1
  Receive/3 -> offset/1
  Receive/2 -> missedData/1

== system acdcmg_sim8_2_sc_gui/OpComm6 ==
  Demux : Demux  Outputs="[1  1  1  3]"
  Receive : opal_lib/Communication/OpRecFromQNX  Node_num=1  Acqu_Group=7  Data_Width=6  Synchronization=on  Interpolation=on  Threshold=1.0  modelname=ACDCMG_sim8.slx  sampletime=4e-05
  busStruct : Subsystem
  dynsig : Terminator
  missedData : Terminator
  offset : Terminator
  samples : Terminator
  sim_time : Terminator
  Out1 : Outport
  Out2 : Outport  Port=2
  Out3 : Outport  Port=3
  Out4 : Outport  Port=4
  wires:
  Demux/4 -> busStruct/4(In4)
  Demux/3 -> busStruct/3(In3)
  Demux/2 -> busStruct/2(In2)
  Demux/1 -> busStruct/1(In1)
  busStruct/4(Out4) -> Out4/1
  busStruct/3(Out3) -> Out3/1
  busStruct/2(Out2) -> Out2/1
  busStruct/1(Out1) -> Out1/1
  Receive/1 -> Demux/1
  Receive/6 -> dynsig/1
  Receive/5 -> samples/1
  Receive/4 -> sim_time/1
  Receive/3 -> offset/1
  Receive/2 -> missedData/1

== system acdcmg_sim8_2_sc_gui/OpComm7 ==
  Demux : Demux  Outputs="[1  1  1  3]"
  Receive : opal_lib/Communication/OpRecFromQNX  Node_num=1  Acqu_Group=8  Data_Width=6  Synchronization=on  Interpolation=on  Threshold=1.0  modelname=ACDCMG_sim8.slx  sampletime=4e-05
  busStruct : Subsystem
  dynsig : Terminator
  missedData : Terminator
  offset : Terminator
  samples : Terminator
  sim_time : Terminator
  Out1 : Outport
  Out2 : Outport  Port=2
  Out3 : Outport  Port=3
  Out4 : Outport  Port=4
  wires:
  Demux/4 -> busStruct/4(In4)
  Demux/3 -> busStruct/3(In3)
  Demux/2 -> busStruct/2(In2)
  Demux/1 -> busStruct/1(In1)
  busStruct/4(Out4) -> Out4/1
  busStruct/3(Out3) -> Out3/1
  busStruct/2(Out2) -> Out2/1
  busStruct/1(Out1) -> Out1/1
  Receive/1 -> Demux/1
  Receive/6 -> dynsig/1
  Receive/5 -> samples/1
  Receive/4 -> sim_time/1
  Receive/3 -> offset/1
  Receive/2 -> missedData/1

== system acdcmg_sim8_2_sc_gui/OpComm8 ==
  Demux : Demux  Outputs="[1  1  3  3]"
  Receive : opal_lib/Communication/OpRecFromQNX  Node_num=1  Acqu_Group=9  Data_Width=8  Synchronization=on  Interpolation=on  Threshold=1.0  modelname=ACDCMG_sim8.slx  sampletime=4e-05
  busStruct : Subsystem
  dynsig : Terminator
  missedData : Terminator
  offset : Terminator
  samples : Terminator
  sim_time : Terminator
  Out1 : Outport
  Out2 : Outport  Port=2
  Out3 : Outport  Port=3
  Out4 : Outport  Port=4
  wires:
  Demux/4 -> busStruct/4(In4)
  Demux/3 -> busStruct/3(In3)
  Demux/2 -> busStruct/2(In2)
  Demux/1 -> busStruct/1(In1)
  busStruct/4(Out4) -> Out4/1
  busStruct/3(Out3) -> Out3/1
  busStruct/2(Out2) -> Out2/1
  busStruct/1(Out1) -> Out1/1
  Receive/1 -> Demux/1
  Receive/6 -> dynsig/1
  Receive/5 -> samples/1
  Receive/4 -> sim_time/1
  Receive/3 -> offset/1
  Receive/2 -> missedData/1

== system acdcmg_sim8_2_sc_gui/OpComm9 ==
  Demux : Demux  Outputs="[1  1  3  3]"
  Receive : opal_lib/Communication/OpRecFromQNX  Node_num=1  Acqu_Group=10  Data_Width=8  Synchronization=on  Interpolation=on  Threshold=1.0  modelname=ACDCMG_sim8.slx  sampletime=4e-05
  busStruct : Subsystem
  dynsig : Terminator
  missedData : Terminator
  offset : Terminator
  samples : Terminator
  sim_time : Terminator
  Out1 : Outport
  Out2 : Outport  Port=2
  Out3 : Outport  Port=3
  Out4 : Outport  Port=4
  wires:
  Demux/4 -> busStruct/4(In4)
  Demux/3 -> busStruct/3(In3)
  Demux/2 -> busStruct/2(In2)
  Demux/1 -> busStruct/1(In1)
  busStruct/4(Out4) -> Out4/1
  busStruct/3(Out3) -> Out3/1
  busStruct/2(Out2) -> Out2/1
  busStruct/1(Out1) -> Out1/1
  Receive/1 -> Demux/1
  Receive/6 -> dynsig/1
  Receive/5 -> samples/1
  Receive/4 -> sim_time/1
  Receive/3 -> offset/1
  Receive/2 -> missedData/1

== system acdcmg_sim8_2_sc_gui/rtlab_send_subsystem ==
  Subsystem23 : Subsystem
  wires:
  [rtlab_send_1] -> Subsystem23/1(In1)
  [rtlab_send_2] -> Subsystem23/2(In2)
  [rtlab_send_3] -> Subsystem23/3(In3)
  [rtlab_send_4] -> Subsystem23/4(In4)
  [rtlab_send_5] -> Subsystem23/5(In5)
  [rtlab_send_6] -> Subsystem23/6(In6)
  [rtlab_send_7] -> Subsystem23/7(In7)
  [rtlab_send_8] -> Subsystem23/8(In8)

== system acdcmg_sim8_2_sc_gui/OpComm/busStruct ==
  In1 : Inport
  In2 : Inport  Port=2
  In3 : Inport  Port=3
  In4 : Inport  Port=4
  Sub1 : Subsystem
  Sub2 : Subsystem
  Sub3 : Subsystem
  Sub4 : Subsystem
  Out1 : Outport
  Out2 : Outport  Port=2
  Out3 : Outport  Port=3
  Out4 : Outport  Port=4
  wires:
  Sub4/1(out) -> Out4/1
  In4/1 -> Sub4/1(in)
  Sub3/1(out) -> Out3/1
  In3/1 -> Sub3/1(in)
  Sub2/1(out) -> Out2/1
  In2/1 -> Sub2/1(in)
  Sub1/1(out) -> Out1/1
  In1/1 -> Sub1/1(in)

== system acdcmg_sim8_2_sc_gui/OpComm1/busStruct ==
  In1 : Inport
  In2 : Inport  Port=2
  In3 : Inport  Port=3
  In4 : Inport  Port=4
  Sub1 : Subsystem
  Sub2 : Subsystem
  Sub3 : Subsystem
  Sub4 : Subsystem
  Out1 : Outport
  Out2 : Outport  Port=2
  Out3 : Outport  Port=3
  Out4 : Outport  Port=4
  wires:
  Sub4/1(out) -> Out4/1
  In4/1 -> Sub4/1(in)
  Sub3/1(out) -> Out3/1
  In3/1 -> Sub3/1(in)
  Sub2/1(out) -> Out2/1
  In2/1 -> Sub2/1(in)
  Sub1/1(out) -> Out1/1
  In1/1 -> Sub1/1(in)

== system acdcmg_sim8_2_sc_gui/OpComm10/busStruct ==
  In1 : Inport
  In2 : Inport  Port=2
  In3 : Inport  Port=3
  In4 : Inport  Port=4
  Sub1 : Subsystem
  Sub2 : Subsystem
  Sub3 : Subsystem
  Sub4 : Subsystem
  Out1 : Outport
  Out2 : Outport  Port=2
  Out3 : Outport  Port=3
  Out4 : Outport  Port=4
  wires:
  Sub4/1(out) -> Out4/1
  In4/1 -> Sub4/1(in)
  Sub3/1(out) -> Out3/1
  In3/1 -> Sub3/1(in)
  Sub2/1(out) -> Out2/1
  In2/1 -> Sub2/1(in)
  Sub1/1(out) -> Out1/1
  In1/1 -> Sub1/1(in)

== system acdcmg_sim8_2_sc_gui/OpComm11/busStruct ==
  In1 : Inport
  In2 : Inport  Port=2
  In3 : Inport  Port=3
  In4 : Inport  Port=4
  Sub1 : Subsystem
  Sub2 : Subsystem
  Sub3 : Subsystem
  Sub4 : Subsystem
  Out1 : Outport
  Out2 : Outport  Port=2
  Out3 : Outport  Port=3
  Out4 : Outport  Port=4
  wires:
  Sub4/1(out) -> Out4/1
  In4/1 -> Sub4/1(in)
  Sub3/1(out) -> Out3/1
  In3/1 -> Sub3/1(in)
  Sub2/1(out) -> Out2/1
  In2/1 -> Sub2/1(in)
  Sub1/1(out) -> Out1/1
  In1/1 -> Sub1/1(in)

== system acdcmg_sim8_2_sc_gui/OpComm12/busStruct ==
  In1 : Inport
  In2 : Inport  Port=2
  In3 : Inport  Port=3
  In4 : Inport  Port=4
  Sub1 : Subsystem
  Sub2 : Subsystem
  Sub3 : Subsystem
  Sub4 : Subsystem
  Out1 : Outport
  Out2 : Outport  Port=2
  Out3 : Outport  Port=3
  Out4 : Outport  Port=4
  wires:
  Sub4/1(out) -> Out4/1
  In4/1 -> Sub4/1(in)
  Sub3/1(out) -> Out3/1
  In3/1 -> Sub3/1(in)
  Sub2/1(out) -> Out2/1
  In2/1 -> Sub2/1(in)
  Sub1/1(out) -> Out1/1
  In1/1 -> Sub1/1(in)

== system acdcmg_sim8_2_sc_gui/OpComm13/busStruct ==
  In1 : Inport
  In2 : Inport  Port=2
  In3 : Inport  Port=3
  In4 : Inport  Port=4
  Sub1 : Subsystem
  Sub2 : Subsystem
  Sub3 : Subsystem
  Sub4 : Subsystem
  Out1 : Outport
  Out2 : Outport  Port=2
  Out3 : Outport  Port=3
  Out4 : Outport  Port=4
  wires:
  Sub4/1(out) -> Out4/1
  In4/1 -> Sub4/1(in)
  Sub3/1(out) -> Out3/1
  In3/1 -> Sub3/1(in)
  Sub2/1(out) -> Out2/1
  In2/1 -> Sub2/1(in)
  Sub1/1(out) -> Out1/1
  In1/1 -> Sub1/1(in)

== system acdcmg_sim8_2_sc_gui/OpComm14/busStruct ==
  In1 : Inport
  In2 : Inport  Port=2
  In3 : Inport  Port=3
  In4 : Inport  Port=4
  Sub1 : Subsystem
  Sub2 : Subsystem
  Sub3 : Subsystem
  Sub4 : Subsystem
  Out1 : Outport
  Out2 : Outport  Port=2
  Out3 : Outport  Port=3
  Out4 : Outport  Port=4
  wires:
  Sub4/1(out) -> Out4/1
  In4/1 -> Sub4/1(in)
  Sub3/1(out) -> Out3/1
  In3/1 -> Sub3/1(in)
  Sub2/1(out) -> Out2/1
  In2/1 -> Sub2/1(in)
  Sub1/1(out) -> Out1/1
  In1/1 -> Sub1/1(in)

== system acdcmg_sim8_2_sc_gui/OpComm15/busStruct ==
  In1 : Inport
  In2 : Inport  Port=2
  In3 : Inport  Port=3
  Sub1 : Subsystem
  Sub2 : Subsystem
  Sub3 : Subsystem
  Out1 : Outport
  Out2 : Outport  Port=2
  Out3 : Outport  Port=3
  wires:
  Sub3/1(out) -> Out3/1
  In3/1 -> Sub3/1(in)
  Sub2/1(out) -> Out2/1
  In2/1 -> Sub2/1(in)
  Sub1/1(out) -> Out1/1
  In1/1 -> Sub1/1(in)

== system acdcmg_sim8_2_sc_gui/OpComm16/busStruct ==
  In1 : Inport
  In2 : Inport  Port=2
  In3 : Inport  Port=3
  In4 : Inport  Port=4
  Sub1 : Subsystem
  Sub2 : Subsystem
  Sub3 : Subsystem
  Sub4 : Subsystem
  Out1 : Outport
  Out2 : Outport  Port=2
  Out3 : Outport  Port=3
  Out4 : Outport  Port=4
  wires:
  Sub4/1(out) -> Out4/1
  In4/1 -> Sub4/1(in)
  Sub3/1(out) -> Out3/1
  In3/1 -> Sub3/1(in)
  Sub2/1(out) -> Out2/1
  In2/1 -> Sub2/1(in)
  Sub1/1(out) -> Out1/1
  In1/1 -> Sub1/1(in)

== system acdcmg_sim8_2_sc_gui/OpComm17/busStruct ==
  In1 : Inport
  In2 : Inport  Port=2
  In3 : Inport  Port=3
  In4 : Inport  Port=4
  Sub1 : Subsystem
  Sub2 : Subsystem
  Sub3 : Subsystem
  Sub4 : Subsystem
  Out1 : Outport
  Out2 : Outport  Port=2
  Out3 : Outport  Port=3
  Out4 : Outport  Port=4
  wires:
  Sub4/1(out) -> Out4/1
  In4/1 -> Sub4/1(in)
  Sub3/1(out) -> Out3/1
  In3/1 -> Sub3/1(in)
  Sub2/1(out) -> Out2/1
  In2/1 -> Sub2/1(in)
  Sub1/1(out) -> Out1/1
  In1/1 -> Sub1/1(in)

== system acdcmg_sim8_2_sc_gui/OpComm18/busStruct ==
  In1 : Inport
  In2 : Inport  Port=2
  In3 : Inport  Port=3
  Sub1 : Subsystem
  Sub2 : Subsystem
  Sub3 : Subsystem
  Out1 : Outport
  Out2 : Outport  Port=2
  Out3 : Outport  Port=3
  wires:
  Sub3/1(out) -> Out3/1
  In3/1 -> Sub3/1(in)
  Sub2/1(out) -> Out2/1
  In2/1 -> Sub2/1(in)
  Sub1/1(out) -> Out1/1
  In1/1 -> Sub1/1(in)

== system acdcmg_sim8_2_sc_gui/OpComm19/busStruct ==
  In1 : Inport
  In2 : Inport  Port=2
  In3 : Inport  Port=3
  In4 : Inport  Port=4
  Sub1 : Subsystem
  Sub2 : Subsystem
  Sub3 : Subsystem
  Sub4 : Subsystem
  Out1 : Outport
  Out2 : Outport  Port=2
  Out3 : Outport  Port=3
  Out4 : Outport  Port=4
  wires:
  Sub4/1(out) -> Out4/1
  In4/1 -> Sub4/1(in)
  Sub3/1(out) -> Out3/1
  In3/1 -> Sub3/1(in)
  Sub2/1(out) -> Out2/1
  In2/1 -> Sub2/1(in)
  Sub1/1(out) -> Out1/1
  In1/1 -> Sub1/1(in)

== system acdcmg_sim8_2_sc_gui/OpComm2/busStruct ==
  In1 : Inport
  In2 : Inport  Port=2
  In3 : Inport  Port=3
  In4 : Inport  Port=4
  Sub1 : Subsystem
  Sub2 : Subsystem
  Sub3 : Subsystem
  Sub4 : Subsystem
  Out1 : Outport
  Out2 : Outport  Port=2
  Out3 : Outport  Port=3
  Out4 : Outport  Port=4
  wires:
  Sub4/1(out) -> Out4/1
  In4/1 -> Sub4/1(in)
  Sub3/1(out) -> Out3/1
  In3/1 -> Sub3/1(in)
  Sub2/1(out) -> Out2/1
  In2/1 -> Sub2/1(in)
  Sub1/1(out) -> Out1/1
  In1/1 -> Sub1/1(in)

== system acdcmg_sim8_2_sc_gui/OpComm20/busStruct ==
  In1 : Inport
  In2 : Inport  Port=2
  In3 : Inport  Port=3
  In4 : Inport  Port=4
  Sub1 : Subsystem
  Sub2 : Subsystem
  Sub3 : Subsystem
  Sub4 : Subsystem
  Out1 : Outport
  Out2 : Outport  Port=2
  Out3 : Outport  Port=3
  Out4 : Outport  Port=4
  wires:
  Sub4/1(out) -> Out4/1
  In4/1 -> Sub4/1(in)
  Sub3/1(out) -> Out3/1
  In3/1 -> Sub3/1(in)
  Sub2/1(out) -> Out2/1
  In2/1 -> Sub2/1(in)
  Sub1/1(out) -> Out1/1
  In1/1 -> Sub1/1(in)

== system acdcmg_sim8_2_sc_gui/OpComm21/busStruct ==
  In1 : Inport
  In2 : Inport  Port=2
  Sub1 : Subsystem
  Sub2 : Subsystem
  Out1 : Outport
  Out2 : Outport  Port=2
  wires:
  Sub2/1(out) -> Out2/1
  In2/1 -> Sub2/1(in)
  Sub1/1(out) -> Out1/1
  In1/1 -> Sub1/1(in)

== system acdcmg_sim8_2_sc_gui/OpComm3/busStruct ==
  In1 : Inport
  In2 : Inport  Port=2
  In3 : Inport  Port=3
  In4 : Inport  Port=4
  Sub1 : Subsystem
  Sub2 : Subsystem
  Sub3 : Subsystem
  Sub4 : Subsystem
  Out1 : Outport
  Out2 : Outport  Port=2
  Out3 : Outport  Port=3
  Out4 : Outport  Port=4
  wires:
  Sub4/1(out) -> Out4/1
  In4/1 -> Sub4/1(in)
  Sub3/1(out) -> Out3/1
  In3/1 -> Sub3/1(in)
  Sub2/1(out) -> Out2/1
  In2/1 -> Sub2/1(in)
  Sub1/1(out) -> Out1/1
  In1/1 -> Sub1/1(in)

== system acdcmg_sim8_2_sc_gui/OpComm4/busStruct ==
  In1 : Inport
  In2 : Inport  Port=2
  In3 : Inport  Port=3
  In4 : Inport  Port=4
  Sub1 : Subsystem
  Sub2 : Subsystem
  Sub3 : Subsystem
  Sub4 : Subsystem
  Out1 : Outport
  Out2 : Outport  Port=2
  Out3 : Outport  Port=3
  Out4 : Outport  Port=4
  wires:
  Sub4/1(out) -> Out4/1
  In4/1 -> Sub4/1(in)
  Sub3/1(out) -> Out3/1
  In3/1 -> Sub3/1(in)
  Sub2/1(out) -> Out2/1
  In2/1 -> Sub2/1(in)
  Sub1/1(out) -> Out1/1
  In1/1 -> Sub1/1(in)

== system acdcmg_sim8_2_sc_gui/OpComm5/busStruct ==
  In1 : Inport
  In2 : Inport  Port=2
  In3 : Inport  Port=3
  In4 : Inport  Port=4
  Sub1 : Subsystem
  Sub2 : Subsystem
  Sub3 : Subsystem
  Sub4 : Subsystem
  Out1 : Outport
  Out2 : Outport  Port=2
  Out3 : Outport  Port=3
  Out4 : Outport  Port=4
  wires:
  Sub4/1(out) -> Out4/1
  In4/1 -> Sub4/1(in)
  Sub3/1(out) -> Out3/1
  In3/1 -> Sub3/1(in)
  Sub2/1(out) -> Out2/1
  In2/1 -> Sub2/1(in)
  Sub1/1(out) -> Out1/1
  In1/1 -> Sub1/1(in)

== system acdcmg_sim8_2_sc_gui/OpComm6/busStruct ==
  In1 : Inport
  In2 : Inport  Port=2
  In3 : Inport  Port=3
  In4 : Inport  Port=4
  Sub1 : Subsystem
  Sub2 : Subsystem
  Sub3 : Subsystem
  Sub4 : Subsystem
  Out1 : Outport
  Out2 : Outport  Port=2
  Out3 : Outport  Port=3
  Out4 : Outport  Port=4
  wires:
  Sub4/1(out) -> Out4/1
  In4/1 -> Sub4/1(in)
  Sub3/1(out) -> Out3/1
  In3/1 -> Sub3/1(in)
  Sub2/1(out) -> Out2/1
  In2/1 -> Sub2/1(in)
  Sub1/1(out) -> Out1/1
  In1/1 -> Sub1/1(in)

== system acdcmg_sim8_2_sc_gui/OpComm7/busStruct ==
  In1 : Inport
  In2 : Inport  Port=2
  In3 : Inport  Port=3
  In4 : Inport  Port=4
  Sub1 : Subsystem
  Sub2 : Subsystem
  Sub3 : Subsystem
  Sub4 : Subsystem
  Out1 : Outport
  Out2 : Outport  Port=2
  Out3 : Outport  Port=3
  Out4 : Outport  Port=4
  wires:
  Sub4/1(out) -> Out4/1
  In4/1 -> Sub4/1(in)
  Sub3/1(out) -> Out3/1
  In3/1 -> Sub3/1(in)
  Sub2/1(out) -> Out2/1
  In2/1 -> Sub2/1(in)
  Sub1/1(out) -> Out1/1
  In1/1 -> Sub1/1(in)

== system acdcmg_sim8_2_sc_gui/OpComm8/busStruct ==
  In1 : Inport
  In2 : Inport  Port=2
  In3 : Inport  Port=3
  In4 : Inport  Port=4
  Sub1 : Subsystem
  Sub2 : Subsystem
  Sub3 : Subsystem
  Sub4 : Subsystem
  Out1 : Outport
  Out2 : Outport  Port=2
  Out3 : Outport  Port=3
  Out4 : Outport  Port=4
  wires:
  Sub4/1(out) -> Out4/1
  In4/1 -> Sub4/1(in)
  Sub3/1(out) -> Out3/1
  In3/1 -> Sub3/1(in)
  Sub2/1(out) -> Out2/1
  In2/1 -> Sub2/1(in)
  Sub1/1(out) -> Out1/1
  In1/1 -> Sub1/1(in)

== system acdcmg_sim8_2_sc_gui/OpComm9/busStruct ==
  In1 : Inport
  In2 : Inport  Port=2
  In3 : Inport  Port=3
  In4 : Inport  Port=4
  Sub1 : Subsystem
  Sub2 : Subsystem
  Sub3 : Subsystem
  Sub4 : Subsystem
  Out1 : Outport
  Out2 : Outport  Port=2
  Out3 : Outport  Port=3
  Out4 : Outport  Port=4
  wires:
  Sub4/1(out) -> Out4/1
  In4/1 -> Sub4/1(in)
  Sub3/1(out) -> Out3/1
  In3/1 -> Sub3/1(in)
  Sub2/1(out) -> Out2/1
  In2/1 -> Sub2/1(in)
  Sub1/1(out) -> Out1/1
  In1/1 -> Sub1/1(in)

== system acdcmg_sim8_2_sc_gui/rtlab_send_subsystem/Subsystem23 ==
  In1 : Inport  PortDimensions=1
  In2 : Inport  Port=2  PortDimensions=1
  In3 : Inport  Port=3  PortDimensions=1
  In4 : Inport  Port=4  PortDimensions=1
  In5 : Inport  Port=5  PortDimensions=1
  In6 : Inport  Port=6  PortDimensions=1
  In7 : Inport  Port=7  PortDimensions=1
  In8 : Inport  Port=8  PortDimensions=1
  Mux : Mux  Inputs=8
  Send23 : opal_lib/Communication/OpSendPar ToQNX  Node_num=1  modelname=ACDCMG_sim8
  wires:
  Mux/1 -> Send23/1
  In1/1 -> Mux/1
  In2/1 -> Mux/2
  In3/1 -> Mux/3
  In4/1 -> Mux/4
  In5/1 -> Mux/5
  In6/1 -> Mux/6
  In7/1 -> Mux/7
  In8/1 -> Mux/8

== system acdcmg_sim8_2_sc_gui/OpComm/busStruct/Sub1 ==
  in : Inport
  out : Outport
  wires:
  in/1 -> out/1  "D_Pa_kW"

== system acdcmg_sim8_2_sc_gui/OpComm/busStruct/Sub2 ==
  in : Inport
  out : Outport
  wires:
  in/1 -> out/1  "D_Pb_kW"

== system acdcmg_sim8_2_sc_gui/OpComm/busStruct/Sub3 ==
  in : Inport
  out : Outport
  wires:
  in/1 -> out/1  "D_Pc_kW"

== system acdcmg_sim8_2_sc_gui/OpComm/busStruct/Sub4 ==
  in : Inport
  out : Outport
  wires:
  in/1 -> out/1  "signal1"

== system acdcmg_sim8_2_sc_gui/OpComm1/busStruct/Sub1 ==
  in : Inport
  out : Outport
  wires:
  in/1 -> out/1  "signal1"

== system acdcmg_sim8_2_sc_gui/OpComm1/busStruct/Sub2 ==
  in : Inport
  out : Outport
  wires:
  in/1 -> out/1  "signal1"

== system acdcmg_sim8_2_sc_gui/OpComm1/busStruct/Sub3 ==
  in : Inport
  out : Outport
  wires:
  in/1 -> out/1  "signal1"

== system acdcmg_sim8_2_sc_gui/OpComm1/busStruct/Sub4 ==
  in : Inport
  out : Outport
  wires:
  in/1 -> out/1  "signal"

== system acdcmg_sim8_2_sc_gui/OpComm10/busStruct/Sub1 ==
  in : Inport
  out : Outport
  wires:
  in/1 -> out/1  "D_Pa_kW"

== system acdcmg_sim8_2_sc_gui/OpComm10/busStruct/Sub2 ==
  in : Inport
  out : Outport
  wires:
  in/1 -> out/1  "D_Pb_kW"

== system acdcmg_sim8_2_sc_gui/OpComm10/busStruct/Sub3 ==
  in : Inport
  out : Outport
  wires:
  in/1 -> out/1  "D_Pc_kW"

== system acdcmg_sim8_2_sc_gui/OpComm10/busStruct/Sub4 ==
  in : Inport
  out : Outport
  wires:
  in/1 -> out/1  "signal1"

== system acdcmg_sim8_2_sc_gui/OpComm11/busStruct/Sub1 ==
  in : Inport
  out : Outport
  wires:
  in/1 -> out/1  "signal1"

== system acdcmg_sim8_2_sc_gui/OpComm11/busStruct/Sub2 ==
  in : Inport
  out : Outport
  wires:
  in/1 -> out/1  "signal1"

== system acdcmg_sim8_2_sc_gui/OpComm11/busStruct/Sub3 ==
  in : Inport
  out : Outport
  wires:
  in/1 -> out/1  "signal1"

== system acdcmg_sim8_2_sc_gui/OpComm11/busStruct/Sub4 ==
  in : Inport
  out : Outport
  wires:
  in/1 -> out/1  "Iabc"

== system acdcmg_sim8_2_sc_gui/OpComm12/busStruct/Sub1 ==
  in : Inport
  out : Outport
  wires:
  in/1 -> out/1  "D_Pa_kW"

== system acdcmg_sim8_2_sc_gui/OpComm12/busStruct/Sub2 ==
  in : Inport
  out : Outport
  wires:
  in/1 -> out/1  "D_Pb_kW"

== system acdcmg_sim8_2_sc_gui/OpComm12/busStruct/Sub3 ==
  in : Inport
  out : Outport
  wires:
  in/1 -> out/1  "D_Pc_kW"

== system acdcmg_sim8_2_sc_gui/OpComm12/busStruct/Sub4 ==
  in : Inport
  out : Outport
  wires:
  in/1 -> out/1  "signal1"

== system acdcmg_sim8_2_sc_gui/OpComm13/busStruct/Sub1 ==
  in : Inport
  out : Outport
  wires:
  in/1 -> out/1  "signal1"

== system acdcmg_sim8_2_sc_gui/OpComm13/busStruct/Sub2 ==
  in : Inport
  out : Outport
  wires:
  in/1 -> out/1  "signal1"

== system acdcmg_sim8_2_sc_gui/OpComm13/busStruct/Sub3 ==
  in : Inport
  out : Outport
  wires:
  in/1 -> out/1  "signal1"

== system acdcmg_sim8_2_sc_gui/OpComm13/busStruct/Sub4 ==
  in : Inport
  out : Outport
  wires:
  in/1 -> out/1  "signal"

== system acdcmg_sim8_2_sc_gui/OpComm14/busStruct/Sub1 ==
  in : Inport
  out : Outport
  wires:
  in/1 -> out/1  "signal1"

== system acdcmg_sim8_2_sc_gui/OpComm14/busStruct/Sub2 ==
  in : Inport
  out : Outport
  wires:
  in/1 -> out/1  "signal1"

== system acdcmg_sim8_2_sc_gui/OpComm14/busStruct/Sub3 ==
  in : Inport
  out : Outport
  wires:
  in/1 -> out/1  "signal1"

== system acdcmg_sim8_2_sc_gui/OpComm14/busStruct/Sub4 ==
  in : Inport
  out : Outport
  wires:
  in/1 -> out/1  "signal1"

== system acdcmg_sim8_2_sc_gui/OpComm15/busStruct/Sub1 ==
  in : Inport
  out : Outport
  wires:
  in/1 -> out/1  "signal1"

== system acdcmg_sim8_2_sc_gui/OpComm15/busStruct/Sub2 ==
  in : Inport
  out : Outport
  wires:
  in/1 -> out/1  "Power (kW)"

== system acdcmg_sim8_2_sc_gui/OpComm15/busStruct/Sub3 ==
  in : Inport
  out : Outport
  wires:
  in/1 -> out/1  "signal1"

== system acdcmg_sim8_2_sc_gui/OpComm16/busStruct/Sub1 ==
  in : Inport
  out : Outport
  wires:
  in/1 -> out/1  "Pmean  (kW)"

== system acdcmg_sim8_2_sc_gui/OpComm16/busStruct/Sub2 ==
  in : Inport
  out : Outport
  wires:
  in/1 -> out/1  "Vmean (V)"

== system acdcmg_sim8_2_sc_gui/OpComm16/busStruct/Sub3 ==
  in : Inport
  out : Outport
  wires:
  in/1 -> out/1  "signal1"

== system acdcmg_sim8_2_sc_gui/OpComm16/busStruct/Sub4 ==
  in : Inport
  out : Outport
  wires:
  in/1 -> out/1  "Irradiance (W/m2)"

== system acdcmg_sim8_2_sc_gui/OpComm17/busStruct/Sub1 ==
  in : Inport
  out : Outport
  wires:
  in/1 -> out/1  "Temperature (deg C)"

== system acdcmg_sim8_2_sc_gui/OpComm17/busStruct/Sub2 ==
  in : Inport
  out : Outport
  wires:
  in/1 -> out/1  "Duty Cycle"

== system acdcmg_sim8_2_sc_gui/OpComm17/busStruct/Sub3 ==
  in : Inport
  out : Outport
  wires:
  in/1 -> out/1  "signal1"

== system acdcmg_sim8_2_sc_gui/OpComm17/busStruct/Sub4 ==
  in : Inport
  out : Outport
  wires:
  in/1 -> out/1  "signal1"

== system acdcmg_sim8_2_sc_gui/OpComm18/busStruct/Sub1 ==
  in : Inport
  out : Outport
  wires:
  in/1 -> out/1  "V_PV"

== system acdcmg_sim8_2_sc_gui/OpComm18/busStruct/Sub2 ==
  in : Inport
  out : Outport
  wires:
  in/1 -> out/1  "I_PV"

== system acdcmg_sim8_2_sc_gui/OpComm18/busStruct/Sub3 ==
  in : Inport
  out : Outport
  wires:
  in/1 -> out/1  "I_diode"

== system acdcmg_sim8_2_sc_gui/OpComm19/busStruct/Sub1 ==
  in : Inport
  out : Outport
  wires:
  in/1 -> out/1  "signal1"

== system acdcmg_sim8_2_sc_gui/OpComm19/busStruct/Sub2 ==
  in : Inport
  out : Outport
  wires:
  in/1 -> out/1  "signal1"

== system acdcmg_sim8_2_sc_gui/OpComm19/busStruct/Sub3 ==
  in : Inport
  out : Outport
  wires:
  in/1 -> out/1  "signal1"

== system acdcmg_sim8_2_sc_gui/OpComm19/busStruct/Sub4 ==
  in : Inport
  out : Outport
  wires:
  in/1 -> out/1  "signal1"
